simulink model "beisp_1"  (Simulink 2.20)
settings: Solver=ode45  StartTime=0.0  StopTime=10.0  RelTol=1e-3  AbsTol=1e-6
settings Model: ConsistencyChecking=off  RTWPlaceOutputsASAP=off

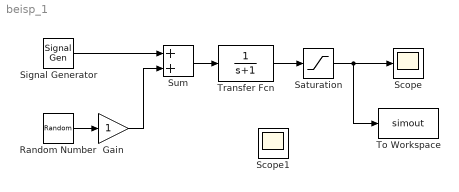
== system beisp_1 ==
  Gain : Gain  Gain=1
  Random Number : RandomNumber  Mean=0  Variance=1  Seed=0  SampleTime=0
  Saturation : Saturate  UpperLimit=4.5  LowerLimit=-4.5
  Scope : Scope
      settings: TickLabels=on  TimeRange=auto  YMin=-5  YMax=5  SaveToWorkspace=off  SaveName=ScopeData
  Scope1 : Scope
      settings: Floating=on  TickLabels=on  TimeRange=auto  YMin=-5  YMax=5  SaveToWorkspace=off  SaveName=ScopeData
  Signal Generator : SignalGenerator  WaveForm=square  Amplitude=5  Frequency=0.15  Units=Hertz
  Sum : Sum  Inputs=++
  To Workspace : ToWorkspace  VariableName=simout  SampleTime=-1
  Transfer Fcn : TransferFcn  Numerator=[1]  Denominator=[1 1]
  wires:
  Random Number/1 -> Gain/1
  Signal Generator/1 -> Sum/1
  Gain/1 -> Sum/2
  Sum/1 -> Transfer Fcn/1
  Transfer Fcn/1 -> Saturation/1
  Saturation/1 -> Scope/1, To Workspace/1
